simulink model "Nanins_LQR_Controller"  (R2015a)
settings: Solver=ode45  StartTime=0.0  StopTime=200  RelTol=1e-3
values from neighbouring files (symbols this model uses):
  A_t = pi*(65/(2*1000))^2    (= 0.00331830724035)    [Nanins_parameters.m]    (also in parameters.m; params.m; systemDynamics.m)
  denorm_t = A_inlet*h_max/t_in    (= 2.36686390533e-06)    [Nanins_parameters.m]
  u0 = ((B_r-W_r)/(2*rho*A_t*g))/h_max    (= 0.226406092405)    [Nanins_parameters.m]
undefined symbols (not defined in the file or in its folder): K
settings Model: CovSFcnEnable=off  Creator=jonas  LastModifiedBy=jonas
settings DataIOCC: LimitDataPoints=off
settings DebuggingCC: SolverPrmCheckMsg=warning

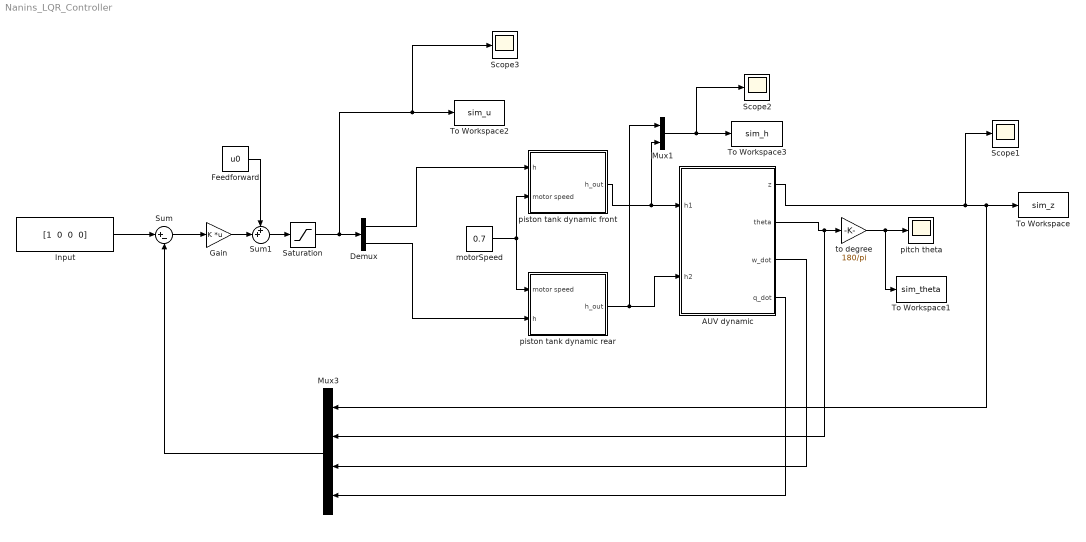
== system Nanins_LQR_Controller ==
  AUV dynamic : Subsystem
  Demux : Demux  Outputs=2
  Feedforward : Constant  Value=u0
  Gain : Gain  Gain=K  Multiplication=Matrix(K*u)
  Input : Constant  Value="[1  0  0  0]"  SampleTime=0.1
  Mux1 : Mux  Inputs=2
  Mux3 : Mux
  Saturation : Saturate  UpperLimit=1  LowerLimit=0
  Scope1 : Scope
  Scope2 : Scope
      settings: SaveName=ScopeData2
  Scope3 : Scope
      settings: SaveName=ScopeData4
  Sum : Sum  Inputs=|+-
  Sum1 : Sum  Inputs=++|
  To Workspace : ToWorkspace  VariableName=sim_z  SampleTime=-1
  To Workspace1 : ToWorkspace  VariableName=sim_theta  SampleTime=-1
  To Workspace2 : ToWorkspace  VariableName=sim_u  SampleTime=-1
  To Workspace3 : ToWorkspace  VariableName=sim_h  SampleTime=-1
  motorSpeed : Constant  Value=0.7
  piston tank dynamic front : Subsystem
  piston tank dynamic rear : Subsystem
  pitch theta : Scope
  to degree : Gain  Gain=180/pi
  wires:
  motorSpeed/1 -> piston tank dynamic front/2(motor speed), piston tank dynamic rear/1(motor speed)
  AUV dynamic/2(theta) -> Mux3/2, to degree/1
  piston tank dynamic front/1(h_out) -> Mux1/2, AUV dynamic/1(h1)
  piston tank dynamic rear/1(h_out) -> Mux1/1, AUV dynamic/2(h2)
  to degree/1 -> To Workspace1/1, pitch theta/1
  Mux1/1 -> Scope2/1, To Workspace3/1
  AUV dynamic/3(w_dot) -> Mux3/3
  AUV dynamic/4(q_dot) -> Mux3/4
  Input/1 -> Sum/1
  Mux3/1 -> Sum/2
  Sum/1 -> Gain/1
  Demux/2 -> piston tank dynamic rear/2(h)
  Demux/1 -> piston tank dynamic front/1(h)
  AUV dynamic/1(z) -> Scope1/1, Mux3/1, To Workspace/1
  Gain/1 -> Sum1/2
  Sum1/1 -> Saturation/1
  Feedforward/1 -> Sum1/1
  Saturation/1 -> Scope3/1, To Workspace2/1, Demux/1

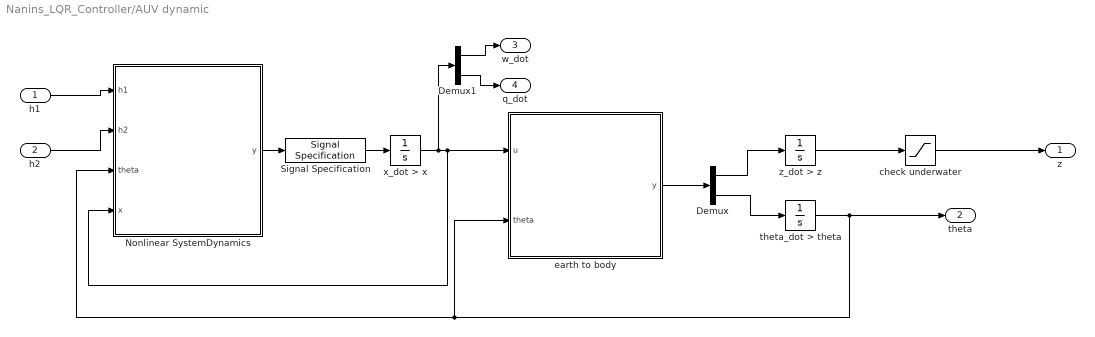
== system Nanins_LQR_Controller/AUV dynamic ==
  h1 : Inport
  h2 : Inport  Port=2
  Demux : Demux  Outputs=2
  Demux1 : Demux  Outputs=2
  Nonlinear SystemDynamics : MATLAB Function  TreatAsAtomicUnit=on
  Signal Specification : SignalSpecification  Dimensions=2
  check underwater : Saturate  UpperLimit=100  LowerLimit=0
  "earth to body " : MATLAB Function  TreatAsAtomicUnit=on
  theta_dot > theta : Integrator  InitialCondition=0.17453
  x_dot > x : Integrator
  z_dot > z : Integrator  InitialCondition=1
  z : Outport
  theta : Outport  Port=2
  w_dot : Outport  Port=3
  q_dot : Outport  Port=4
  wires:
  h2/1 -> Nonlinear SystemDynamics/2(h2)
  Demux/2 -> theta_dot > theta/1
  x_dot > x/1 -> Demux1/1, Nonlinear SystemDynamics/4(x), "earth to body "/1(u)
  h1/1 -> Nonlinear SystemDynamics/1(h1)
  theta_dot > theta/1 -> theta/1, Nonlinear SystemDynamics/3(theta), "earth to body "/2(theta)
  Demux/1 -> z_dot > z/1
  z_dot > z/1 -> check underwater/1
  "earth to body "/1(y) -> Demux/1
  Nonlinear SystemDynamics/1(y) -> Signal Specification/1
  Signal Specification/1 -> x_dot > x/1
  check underwater/1 -> z/1
  Demux1/1 -> w_dot/1
  Demux1/2 -> q_dot/1

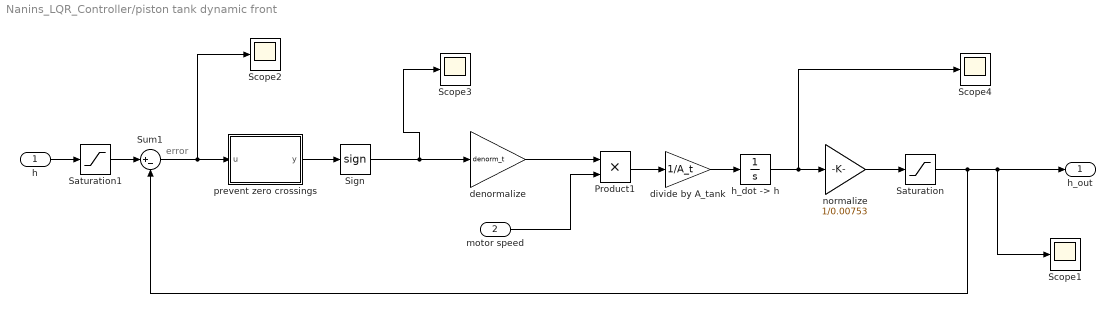
== system Nanins_LQR_Controller/piston tank dynamic front ==
  note: error
  h : Inport
  motor speed : Inport  Port=2
  Product1 : Product
  Saturation : Saturate  UpperLimit=1  LowerLimit=0
  Saturation1 : Saturate  UpperLimit=1  LowerLimit=0
  Scope{1..4} (4 alike) : Scope
      Scope1 settings: SaveName=ScopeData7
      Scope2 settings: SaveName=ScopeData9
      Scope3 settings: SaveName=ScopeData10
      Scope4 settings: SaveName=ScopeData6
  Sign : Signum  ZeroCross=off
  Sum1 : Sum  Inputs=|+-
  denormalize : Gain  Gain=denorm_t
  divide by A_tank : Gain  Gain=1/A_t
  "h_dot -> h" : Integrator  InitialCondition=0.0017057  UpperSaturationLimit=1  LowerSaturationLimit=0
  normalize : Gain  Gain=1/0.00753
  prevent zero crossings : MATLAB Function  TreatAsAtomicUnit=on
  h_out : Outport
  wires:
  Saturation/1 -> h_out/1, Scope1/1, Sum1/2
  normalize/1 -> Saturation/1
  "h_dot -> h"/1 -> Scope4/1, normalize/1
  divide by A_tank/1 -> "h_dot -> h"/1
  h/1 -> Saturation1/1
  denormalize/1 -> Product1/1
  motor speed/1 -> Product1/2
  Product1/1 -> divide by A_tank/1
  Sum1/1 -> prevent zero crossings/1(u), Scope2/1
  Sign/1 -> Scope3/1, denormalize/1
  prevent zero crossings/1(y) -> Sign/1
  Saturation1/1 -> Sum1/1

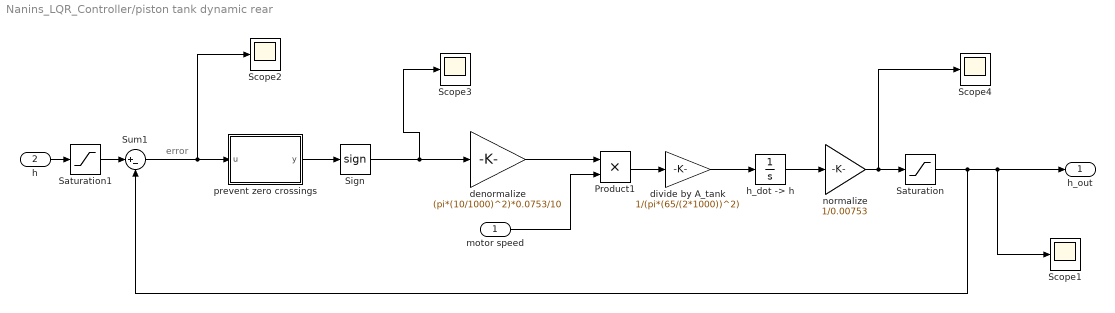
== system Nanins_LQR_Controller/piston tank dynamic rear ==
  note: error
  motor speed : Inport
  h : Inport  Port=2
  Product1 : Product
  Saturation : Saturate  UpperLimit=1  LowerLimit=0
  Saturation1 : Saturate  UpperLimit=1  LowerLimit=0
  Scope{1..4} (4 alike) : Scope
      Scope1 settings: SaveName=ScopeData7
      Scope2 settings: SaveName=ScopeData9
      Scope3 settings: SaveName=ScopeData10
      Scope4 settings: SaveName=ScopeData6
  Sign : Signum  ZeroCross=off
  Sum1 : Sum  Inputs=|+-
  denormalize : Gain  Gain=(pi*(10/1000)^2)*0.0753/10
  divide by A_tank : Gain  Gain=1/(pi*(65/(2*1000))^2)
  "h_dot -> h" : Integrator  InitialCondition=0.0017057  UpperSaturationLimit=1  LowerSaturationLimit=0
  normalize : Gain  Gain=1/0.00753
  prevent zero crossings : MATLAB Function  TreatAsAtomicUnit=on
  h_out : Outport
  wires:
  prevent zero crossings/1(y) -> Sign/1
  Sign/1 -> denormalize/1, Scope3/1
  Sum1/1 -> Scope2/1, prevent zero crossings/1(u)
  Product1/1 -> divide by A_tank/1
  motor speed/1 -> Product1/2
  denormalize/1 -> Product1/1
  h/1 -> Saturation1/1
  divide by A_tank/1 -> "h_dot -> h"/1
  "h_dot -> h"/1 -> normalize/1
  normalize/1 -> Saturation/1, Scope4/1
  Saturation/1 -> Sum1/2, Scope1/1, h_out/1
  Saturation1/1 -> Sum1/1

== matlab function Nanins_LQR_Controller/AUV dynamic/earth to body  ==
  data: u input; y output; theta input
function y = fcn(u, theta)
%#codegen
x = u;

J = [cos(theta), 0;
    0, 1];

y = J*x;

== matlab function Nanins_LQR_Controller/AUV dynamic/Nonlinear SystemDynamics ==
  data: h1 input; y output; h2 input; theta input; x input
function y = fcn(h1, h2, theta, x)
%#codegen

% ---- PARAMETERS --

g   = 9.81;                 % [m/s^2]   gravity
rho = 1000;                 % [kg/m^3]  density water

% parameters nanins specific
m0  = 5.7;                    % [kg]      empty weight Nanin
l_n = 0.514;                  % [m]       length Nanin
r_n = 0.06;                  % [m]       radius Nanin
V_n = r_n^2*pi*l_n;         % [m^3]     volume Nanin

x0_t = 0.25;                % [m]       displacement piston tank in x direction
z0_t = 0.05;                % [m]       displacement piston tank in z direction
A_t = pi*(65/(2*1000))^2;   % [m^2]     area piston tank
V_t = 250e-6;               % [m^3]     volume of piston tank
h_max = V_t/A_t;            % [m]       max height of water in piston tank

Iy0 = 0.134;                % [kgm^2]   moment of inertia around y-axis

% restoring static forces
W_r = m0*g;          % [N]       gravitational force empty
B_r = rho*g*V_n;    % [N]       buoancy restoring force

% Added mass coefficents
Z_w = -rho*V_n;             % [kg]
M_q = -1/12*rho*V_n*l_n;    % [km*m]

% ------

% Denormalize input
h1 = h1*h_max;
h2 = h2*h_max;

u_vec = [h1; h2];

% calculate dynamic parameters
m = m0 + rho*A_t*(h1+h2); % dynamic mass
x1 = x0_t - h1/2;         % CoG of piston tank
x2 = -(x0_t - h2/2);
X_u = -0.1*m;

z_g = 0.005;
x_g = 0;
I_y = Iy0;

% system matrices

M = [m-Z_w, -m*x_g;...
    -m*x_g, I_y-M_q];

g_static = [-(W_r - B_r)*cos(theta);
            z_g*W_r*sin(theta)+x_g*W_r*cos(theta)];

%g_static = [-(W_r - B_r);
%            x_g*W_r];
        
K = rho*g*A_t*[-cos(theta), -cos(theta);
                sin(theta)*z0_t+cos(theta)*x1, sin(theta)*z0_t+cos(theta)*x2];

D = -diag([Z_w*abs(x(1)), M_q*abs(x(2))]);
%D = zeros(2,2);

%K = rho*g*A_t*[-1, -1;
%                x1, x2];
            
% calculate state

x_dot = M\(-D*x-K*u_vec - g_static);

y = x_dot;

== matlab function Nanins_LQR_Controller/piston tank dynamic front/prevent zero crossings ==
  data: u input; y output
function y = fcn(u)
%#codegen

threshhold = 0.005;

if(abs(u)<threshhold)
    out = 0;
else 
    out = u;
end

y = out;

== matlab function Nanins_LQR_Controller/piston tank dynamic rear/prevent zero crossings ==
  data: u input; y output
function y = fcn(u)
%#codegen

threshhold = 0.005;

if(abs(u)<threshhold)
    out = 0;
else 
    out = u;
end

y = out;
